simulink model "quadrotor_multibody_plant"  (R2026a)
settings: Solver=ode4  StopTime=5  FixedStep=0.002
settings Model: Creator=bettim  LastModifiedBy=bettim

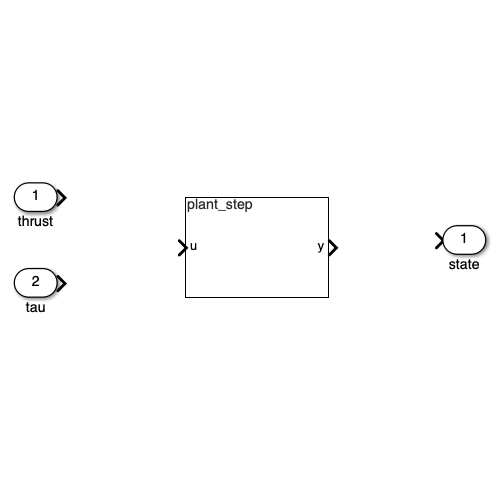
[thumbnail: Simulink's stored preview of the top-level diagram]
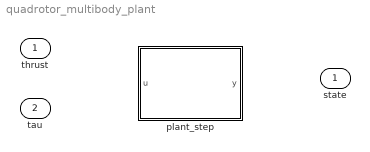
== system quadrotor_multibody_plant ==
  thrust : Inport
  tau : Inport  Port=2
  plant_step : MATLAB Function  TreatAsAtomicUnit=on
  state : Outport

== matlab function quadrotor_multibody_plant/plant_step ==
  data: u input; y output
function y = fcn(u)

y = u;
